simulink model "IB_BIEN_y_TG_BIEN"  (Simulink 8.1)
settings: Solver=ode45  StartTime=0.0  StopTime=50  RelTol=1e-3
PreLoadFcn:
  | Initial_datab
  | Const_IB
values from neighbouring files (symbols this model uses):
  a1 = (Iyy-Izz)/Ixx    (= -1.125)    [Initial_datab.m]
  a2 = Jr/Ixx    (= 0.00697115384615)    [Initial_datab.m]
  a3 = (Izz-Ixx)/Iyy    (= 1.11607142857)    [Initial_datab.m]
  a5 = (Ixx-Iyy)/Izz    (= -0.0349344978166)    [Initial_datab.m]
  alp1 = 20    [Initial_datab.m]
  alp2 = 10    [Initial_datab.m]
  b = 1.2*10^(-4)    (= 0.00012)    [Initial_datab.m]
  b1 = 1/Ixx    (= 96.1538461538)    [Initial_datab.m]
  b2 = 1/Iyy    (= 89.2857142857)    [Initial_datab.m]
  b3 = 1/Izz    (= 43.6681222707)    [Initial_datab.m]
  c1 = 10    [Const_IB.m]
  c10 = 0.75    [Const_IB.m]
  c11 = 1    [Const_IB.m]
  c12 = 0.75    [Const_IB.m]
  c2 = 6    [Const_IB.m]
  c3 = 10    [Const_IB.m]
  c4 = 6    [Const_IB.m]
  c5 = 2    [Const_IB.m]
  c6 = 2    [Const_IB.m]
  c7 = 3.5    [Const_IB.m]
  c8 = 1.5    [Const_IB.m]
  c9 = 1    [Const_IB.m]
  d = 3*10^(-6)    (= 3e-06)    [Initial_datab.m]
  Ixx = 10.4*10^(-3)    (= 0.0104)    [Initial_datab.m]
  Iyy = 11.2*10^(-3)    (= 0.0112)    [Initial_datab.m]
  Izz = 2.29*10^(-2)    (= 0.0229)    [Initial_datab.m]
  Jr = 7.25*10^(-5)    (= 7.25e-05)    [Initial_datab.m]
  k1x = -k1x    (= -0.5)    [Initial_datab.m]
  k1y = -k1y    (= -0.5)    [Initial_datab.m]
  k1z = -k1z    (= -2)    [Initial_datab.m]
  l = 0.225    [Initial_datab.m]
  ld1 = 0.07    [Const_IB.m]
  ld2 = 0.05    [Const_IB.m]
  ld3 = 0.01    [Const_IB.m]
  ld4 = 0.01    [Const_IB.m]
  ld5 = 0.001    [Const_IB.m]
  ld6 = 0.001    [Const_IB.m]
  m = 1.14    [Initial_datab.m]
  phi0 = 0    [Initial_datab.m]
  phi0dot = 0    [Initial_datab.m]
  psi0 = 0    [Initial_datab.m]
  psi0dot = 0    [Initial_datab.m]
  theta0 = 0    [Initial_datab.m]
  theta0dot = 0    [Initial_datab.m]
  x0 = 0    [Initial_datab.m]
  x0dot = 0    [Initial_datab.m]
  xf = -5    [Initial_datab.m]
  xfdot = 0    [Initial_datab.m]
  y0 = 0    [Initial_datab.m]
  y0dot = 0    [Initial_datab.m]
  yf = 5    [Initial_datab.m]
  yfdot = 0    [Initial_datab.m]
  z0 = 0    [Initial_datab.m]
  z0dot = 0    [Initial_datab.m]
  zf = 50    [Initial_datab.m]
  zfdot = 0    [Initial_datab.m]
undefined symbols (not defined in the file or in its folder): sigbuilder_block
(part 2 of 2)

== system IB_BIEN_y_TG_BIEN/TRAJECTORY GENERATION/Subsystem5/Subsystem1 ==
  t : Inport
  In2 : Inport  Port=2
  y_ent0 : Inport  Port=3
  Enabled Subsystem : Subsystem  TreatAsAtomicUnit=on
  Enabled Subsystem1 : Subsystem  TreatAsAtomicUnit=on
  Merge : Merge
  Relational Operator : RelationalOperator  Operator===  OutDataTypeStr=boolean
  Relational Operator1 : RelationalOperator  Operator=~=  OutDataTypeStr=boolean
  y0 : Outport
  wires:
  t/1 -> Relational Operator1/1, Relational Operator/1
  In2/1 -> Relational Operator/2, Relational Operator1/2, Enabled Subsystem1/1(In1)
  Relational Operator/1 -> Enabled Subsystem/Enable
  Enabled Subsystem/1(Out1) -> Merge/1
  Relational Operator1/1 -> Enabled Subsystem1/Enable
  Enabled Subsystem1/1(Out1) -> Merge/2
  y_ent0/1 -> Enabled Subsystem/1(In1)
  Merge/1 -> y0/1

== system IB_BIEN_y_TG_BIEN/TRAJECTORY GENERATION/Subsystem5/Subsystem2 ==
  t : Inport
  In2 : Inport  Port=2
  z_ent0 : Inport  Port=3
  Enabled Subsystem : Subsystem  TreatAsAtomicUnit=on
  Enabled Subsystem1 : Subsystem  TreatAsAtomicUnit=on
  Merge : Merge
  Relational Operator : RelationalOperator  Operator===  OutDataTypeStr=boolean
  Relational Operator1 : RelationalOperator  Operator=~=  OutDataTypeStr=boolean
  z0 : Outport
  wires:
  t/1 -> Relational Operator1/1, Relational Operator/1
  In2/1 -> Relational Operator/2, Relational Operator1/2, Enabled Subsystem1/1(In1)
  Relational Operator/1 -> Enabled Subsystem/Enable
  Enabled Subsystem/1(Out1) -> Merge/1
  Relational Operator1/1 -> Enabled Subsystem1/Enable
  Enabled Subsystem1/1(Out1) -> Merge/2
  z_ent0/1 -> Enabled Subsystem/1(In1)
  Merge/1 -> z0/1

== system IB_BIEN_y_TG_BIEN/TRAJECTORY GENERATION/X POSITION/Enabled Subsystem ==
  In1 : Inport
  Enable : EnablePort
  Fcn : Fcn  Expr=u(1)*u(2)+u(3)
  Out1 : Outport
  wires:
  In1/1 -> Fcn/1
  Fcn/1 -> Out1/1

== system IB_BIEN_y_TG_BIEN/TRAJECTORY GENERATION/X POSITION/Enabled Subsystem1 ==
  In1 : Inport
  Enable : EnablePort
  Fcn : Fcn  Expr=u(4)
  Out1 : Outport
  wires:
  In1/1 -> Fcn/1
  Fcn/1 -> Out1/1

== system IB_BIEN_y_TG_BIEN/TRAJECTORY GENERATION/X POSITION/Enabled Subsystem2 ==
  In1 : Inport
  Enable : EnablePort
  Fcn : Fcn  Expr=u(7)*(u(2)-u(5))+u(6)
  Out1 : Outport
  wires:
  In1/1 -> Fcn/1
  Fcn/1 -> Out1/1

== system IB_BIEN_y_TG_BIEN/TRAJECTORY GENERATION/X POSITION/Enabled Subsystem3 ==
  In1 : Inport
  Enable : EnablePort
  Fcn : Fcn  Expr=u(6)
  Out1 : Outport
  wires:
  In1/1 -> Fcn/1
  Fcn/1 -> Out1/1

== system IB_BIEN_y_TG_BIEN/TRAJECTORY GENERATION/X POSITION/Subsystem ==
  x0dot : Inport
  k1x : Inport  Port=2
  Vxmax : Inport  Port=3
  Add1 : Sum  Inputs=+-
  Divide : Product  Inputs=*/
  T1x : Outport
  wires:
  Vxmax/1 -> Add1/1  "Vxmax"
  Add1/1 -> Divide/1
  x0dot/1 -> Add1/2
  Divide/1 -> T1x/1  "T1"
  k1x/1 -> Divide/2

== system IB_BIEN_y_TG_BIEN/TRAJECTORY GENERATION/X POSITION/Subsystem1 ==
  deltax : Inport
  x0dot : Inport  Port=2
  k1x : Inport  Port=3
  xfdot : Inport  Port=4
  k2x : Inport  Port=5
  Vxmax : Inport  Port=6
  Add2 : Sum  Inputs=+--++
  Divide1 : Product  Inputs=*/
  Fcn : Fcn  Expr=((u(1)^2)-(u(2)^2))/(2*u(3)*u(1))
  Fcn1 : Fcn  Expr=(u(1)-u(2))/u(3)
  Fcn2 : Fcn  Expr=(u(1)-u(2))/u(3)
  Fcn3 : Fcn  Expr=((u(1)^2)-(u(2)^2))/(2*u(3)*u(1))
  Mux{,1..3} (4 alike) : Mux  Inputs=3
  Tx : Outport
  wires:
  Vxmax/1 -> Divide1/2, Mux/1, Mux1/1, Mux2/1, Mux3/1  "Vxmax"
  deltax/1 -> Divide1/1  "deltax"
  x0dot/1 -> Mux/2, Mux2/2
  k1x/1 -> Mux/3, Mux2/3
  Add2/1 -> Tx/1
  Divide1/1 -> Add2/1
  Mux/1 -> Fcn/1
  Fcn/1 -> Add2/2
  Mux1/1 -> Fcn1/1
  Fcn1/1 -> Add2/3
  Mux2/1 -> Fcn2/1
  Fcn2/1 -> Add2/4
  Mux3/1 -> Fcn3/1
  Fcn3/1 -> Add2/5
  xfdot/1 -> Mux1/2, Mux3/2
  k2x/1 -> Mux3/3, Mux1/3

== system IB_BIEN_y_TG_BIEN/TRAJECTORY GENERATION/X POSITION/Subsystem2 ==
  T : Inport
  xfdot : Inport  Port=2
  k2x : Inport  Port=3
  Vxmax : Inport  Port=4
  Add1 : Sum  Inputs=+-
  Add2 : Sum
  Display{1..4} (4 alike) : Display
  Divide : Product  Inputs=*/
  T2x : Outport
  wires:
  Vxmax/1 -> Add1/1, Display2/1  "Vxmax"
  Add1/1 -> Divide/1
  xfdot/1 -> Add1/2
  k2x/1 -> Divide/2, Display3/1
  Divide/1 -> Add2/1, Display1/1
  T/1 -> Add2/2, Display4/1
  Add2/1 -> T2x/1

== system IB_BIEN_y_TG_BIEN/TRAJECTORY GENERATION/X POSITION/Subsystem3 ==
  t : Inport
  T1 : Inport  Port=2
  T : Inport  Port=3
  T2 : Inport  Port=4
  Logical Operator : Logic  AllPortsSameDT=off  OutDataTypeStr=boolean
  Logical Operator1 : Logic  AllPortsSameDT=off  OutDataTypeStr=boolean
  Relational Operator : RelationalOperator  Operator=<  OutDataTypeStr=boolean
  Relational Operator1 : RelationalOperator  OutDataTypeStr=boolean
  Relational Operator2 : RelationalOperator  Operator=<  OutDataTypeStr=boolean
  Relational Operator3 : RelationalOperator  Operator=<  OutDataTypeStr=boolean
  Relational Operator4 : RelationalOperator  OutDataTypeStr=boolean
  Relational Operator5 : RelationalOperator  OutDataTypeStr=boolean
  Out1 : Outport
  Out2 : Outport  Port=2
  Out3 : Outport  Port=3
  Out4 : Outport  Port=4
  wires:
  T1/1 -> Relational Operator1/2, Relational Operator/2
  T2/1 -> Relational Operator4/2, Relational Operator2/2
  Relational Operator1/1 -> Logical Operator/1
  Relational Operator2/1 -> Logical Operator/2
  Relational Operator3/1 -> Logical Operator1/1
  Relational Operator4/1 -> Logical Operator1/2
  t/1 -> Relational Operator1/1, Relational Operator2/1, Relational Operator3/1, Relational Operator4/1, Relational Operator5/1, Relational Operator/1
  T/1 -> Relational Operator3/2, Relational Operator5/2
  Relational Operator/1 -> Out1/1
  Logical Operator/1 -> Out2/1
  Logical Operator1/1 -> Out3/1
  Relational Operator5/1 -> Out4/1

== system IB_BIEN_y_TG_BIEN/TRAJECTORY GENERATION/X POSITION/Subsystem5 ==
  t : Inport
  T : Inport  Port=2
  k1 : Inport  Port=3
  Fcn3 : Fcn  Expr=u(3)*(1-exp(-alp2*abs(u(1)-u(2))))
  Gain2 : Gain  Gain=-(1/4)
  Mux2 : Mux  Inputs=3
  k2xapro : Outport
  wires:
  Mux2/1 -> Fcn3/1
  Gain2/1 -> Mux2/3  "k2"
  t/1 -> Mux2/1
  T/1 -> Mux2/2
  k1/1 -> Gain2/1
  Fcn3/1 -> k2xapro/1  "k2x_apro"

== system IB_BIEN_y_TG_BIEN/TRAJECTORY GENERATION/Y POSITION/Enabled Subsystem ==
  In1 : Inport
  Enable : EnablePort
  Fcn : Fcn  Expr=u(1)*u(2)+u(3)
  Out1 : Outport
  wires:
  In1/1 -> Fcn/1
  Fcn/1 -> Out1/1

== system IB_BIEN_y_TG_BIEN/TRAJECTORY GENERATION/Y POSITION/Enabled Subsystem1 ==
  In1 : Inport
  Enable : EnablePort
  Fcn : Fcn  Expr=u(4)
  Out1 : Outport
  wires:
  In1/1 -> Fcn/1
  Fcn/1 -> Out1/1

== system IB_BIEN_y_TG_BIEN/TRAJECTORY GENERATION/Y POSITION/Enabled Subsystem2 ==
  In1 : Inport
  Enable : EnablePort
  Fcn : Fcn  Expr=u(7)*(u(2)-u(5))+u(6)
  Out1 : Outport
  wires:
  In1/1 -> Fcn/1
  Fcn/1 -> Out1/1

== system IB_BIEN_y_TG_BIEN/TRAJECTORY GENERATION/Y POSITION/Enabled Subsystem3 ==
  In1 : Inport
  Enable : EnablePort
  Fcn : Fcn  Expr=u(6)
  Out1 : Outport
  wires:
  In1/1 -> Fcn/1
  Fcn/1 -> Out1/1

== system IB_BIEN_y_TG_BIEN/TRAJECTORY GENERATION/Y POSITION/Subsystem ==
  y0dot : Inport
  k1y : Inport  Port=2
  Vymax : Inport  Port=3
  Add1 : Sum  Inputs=+-
  Divide : Product  Inputs=*/
  T1y : Outport
  wires:
  Vymax/1 -> Add1/1  "Vxmax"
  Add1/1 -> Divide/1
  y0dot/1 -> Add1/2
  Divide/1 -> T1y/1  "T1"
  k1y/1 -> Divide/2

== system IB_BIEN_y_TG_BIEN/TRAJECTORY GENERATION/Y POSITION/Subsystem1 ==
  yf : Inport
  y0 : Inport  Port=2
  y0dot : Inport  Port=3
  k1y : Inport  Port=4
  yfdot : Inport  Port=5
  k2y : Inport  Port=6
  Vymax : Inport  Port=7
  Add : Sum  Inputs=+-
  Add2 : Sum  Inputs=+--++
  Divide1 : Product  Inputs=*/
  Fcn : Fcn  Expr=((u(1)^2)-(u(2)^2))/(2*u(3)*u(1))
  Fcn1 : Fcn  Expr=(u(1)-u(2))/u(3)
  Fcn2 : Fcn  Expr=(u(1)-u(2))/u(3)
  Fcn3 : Fcn  Expr=((u(1)^2)-(u(2)^2))/(2*u(3)*u(1))
  Mux{,1..3} (4 alike) : Mux  Inputs=3
  Ty : Outport
  wires:
  Add/1 -> Divide1/1  "deltay"
  Vymax/1 -> Divide1/2, Mux/1, Mux1/1, Mux2/1, Mux3/1  "Vymax"
  yf/1 -> Add/1
  y0/1 -> Add/2
  y0dot/1 -> Mux/2, Mux2/2
  k1y/1 -> Mux/3, Mux2/3
  Add2/1 -> Ty/1
  Divide1/1 -> Add2/1
  Mux/1 -> Fcn/1
  Fcn/1 -> Add2/2
  Mux1/1 -> Fcn1/1
  Fcn1/1 -> Add2/3
  Mux2/1 -> Fcn2/1
  Fcn2/1 -> Add2/4
  Mux3/1 -> Fcn3/1
  Fcn3/1 -> Add2/5
  yfdot/1 -> Mux1/2, Mux3/2
  k2y/1 -> Mux3/3, Mux1/3

== system IB_BIEN_y_TG_BIEN/TRAJECTORY GENERATION/Y POSITION/Subsystem2 ==
  T : Inport
  yfdot : Inport  Port=2
  k2y : Inport  Port=3
  Vymax : Inport  Port=4
  Add1 : Sum  Inputs=+-
  Add2 : Sum
  Divide : Product  Inputs=*/
  T2y : Outport
  wires:
  Vymax/1 -> Add1/1  "Vymax"
  Add1/1 -> Divide/1
  yfdot/1 -> Add1/2
  k2y/1 -> Divide/2
  Divide/1 -> Add2/1
  T/1 -> Add2/2
  Add2/1 -> T2y/1

== system IB_BIEN_y_TG_BIEN/TRAJECTORY GENERATION/Y POSITION/Subsystem3 ==
  t : Inport
  T1 : Inport  Port=2
  T : Inport  Port=3
  T2 : Inport  Port=4
  Logical Operator : Logic  AllPortsSameDT=off  OutDataTypeStr=boolean
  Logical Operator1 : Logic  AllPortsSameDT=off  OutDataTypeStr=boolean
  Relational Operator : RelationalOperator  Operator=<  OutDataTypeStr=boolean
  Relational Operator1 : RelationalOperator  OutDataTypeStr=boolean
  Relational Operator2 : RelationalOperator  Operator=<  OutDataTypeStr=boolean
  Relational Operator3 : RelationalOperator  Operator=<  OutDataTypeStr=boolean
  Relational Operator4 : RelationalOperator  OutDataTypeStr=boolean
  Relational Operator5 : RelationalOperator  OutDataTypeStr=boolean
  Out1 : Outport
  Out2 : Outport  Port=2
  Out3 : Outport  Port=3
  Out4 : Outport  Port=4
  wires:
  T1/1 -> Relational Operator1/2, Relational Operator/2
  T2/1 -> Relational Operator4/2, Relational Operator2/2
  Relational Operator1/1 -> Logical Operator/1
  Relational Operator2/1 -> Logical Operator/2
  Relational Operator3/1 -> Logical Operator1/1
  Relational Operator4/1 -> Logical Operator1/2
  t/1 -> Relational Operator1/1, Relational Operator2/1, Relational Operator3/1, Relational Operator4/1, Relational Operator5/1, Relational Operator/1
  T/1 -> Relational Operator3/2, Relational Operator5/2
  Relational Operator/1 -> Out1/1
  Logical Operator/1 -> Out2/1
  Logical Operator1/1 -> Out3/1
  Relational Operator5/1 -> Out4/1

== system IB_BIEN_y_TG_BIEN/TRAJECTORY GENERATION/Z POSITION/Enabled Subsystem ==
  In1 : Inport
  Enable : EnablePort
  Fcn : Fcn  Expr=u(1)*u(2)+u(3)
  Out1 : Outport
  wires:
  In1/1 -> Fcn/1
  Fcn/1 -> Out1/1

== system IB_BIEN_y_TG_BIEN/TRAJECTORY GENERATION/Z POSITION/Enabled Subsystem1 ==
  In1 : Inport
  Enable : EnablePort
  Fcn : Fcn  Expr=u(4)
  Out1 : Outport
  wires:
  In1/1 -> Fcn/1
  Fcn/1 -> Out1/1

== system IB_BIEN_y_TG_BIEN/TRAJECTORY GENERATION/Z POSITION/Enabled Subsystem2 ==
  In1 : Inport
  Enable : EnablePort
  Fcn : Fcn  Expr=u(7)*(u(2)-u(5))+u(6)
  Out1 : Outport
  wires:
  In1/1 -> Fcn/1
  Fcn/1 -> Out1/1

== system IB_BIEN_y_TG_BIEN/TRAJECTORY GENERATION/Z POSITION/Enabled Subsystem3 ==
  In1 : Inport
  Enable : EnablePort
  Fcn : Fcn  Expr=u(6)
  Out1 : Outport
  wires:
  In1/1 -> Fcn/1
  Fcn/1 -> Out1/1

== system IB_BIEN_y_TG_BIEN/TRAJECTORY GENERATION/Z POSITION/Subsystem ==
  z0dot : Inport
  k1z : Inport  Port=2
  Vzmax : Inport  Port=3
  Add1 : Sum  Inputs=+-
  Divide : Product  Inputs=*/
  T1 : Outport
  wires:
  Vzmax/1 -> Add1/1  "Vxmax"
  Add1/1 -> Divide/1
  z0dot/1 -> Add1/2
  Divide/1 -> T1/1  "T1"
  k1z/1 -> Divide/2

== system IB_BIEN_y_TG_BIEN/TRAJECTORY GENERATION/Z POSITION/Subsystem1 ==
  zf : Inport
  z0 : Inport  Port=2
  z0dot : Inport  Port=3
  k1z : Inport  Port=4
  zfdot : Inport  Port=5
  k2z : Inport  Port=6
  Vzmax : Inport  Port=7
  Add : Sum  Inputs=+-
  Add2 : Sum  Inputs=+--++
  Divide1 : Product  Inputs=*/
  Fcn : Fcn  Expr=((u(1)^2)-(u(2)^2))/(2*u(3)*u(1))
  Fcn1 : Fcn  Expr=(u(1)-u(2))/u(3)
  Fcn2 : Fcn  Expr=(u(1)-u(2))/u(3)
  Fcn3 : Fcn  Expr=((u(1)^2)-(u(2)^2))/(2*u(3)*u(1))
  Mux{,1..3} (4 alike) : Mux  Inputs=3
  T : Outport
  wires:
  Add/1 -> Divide1/1  "deltaz"
  zf/1 -> Add/1
  z0/1 -> Add/2
  z0dot/1 -> Mux/2, Mux2/2
  k1z/1 -> Mux/3, Mux2/3
  Add2/1 -> T/1
  Divide1/1 -> Add2/1
  Mux/1 -> Fcn/1
  Fcn/1 -> Add2/2
  Mux1/1 -> Fcn1/1
  Fcn1/1 -> Add2/3
  Mux2/1 -> Fcn2/1
  Fcn2/1 -> Add2/4
  Mux3/1 -> Fcn3/1
  Fcn3/1 -> Add2/5
  zfdot/1 -> Mux1/2, Mux3/2
  k2z/1 -> Mux3/3, Mux1/3
  Vzmax/1 -> Divide1/2, Mux/1, Mux1/1, Mux2/1, Mux3/1  "Vzmax"

== system IB_BIEN_y_TG_BIEN/TRAJECTORY GENERATION/Z POSITION/Subsystem2 ==
  T : Inport
  zfdot : Inport  Port=2
  k2z : Inport  Port=3
  Vzmax : Inport  Port=4
  Add1 : Sum  Inputs=+-
  Add2 : Sum
  Divide : Product  Inputs=*/
  T2 : Outport
  wires:
  Vzmax/1 -> Add1/1  "Vzmax"
  Add1/1 -> Divide/1
  zfdot/1 -> Add1/2
  k2z/1 -> Divide/2
  Divide/1 -> Add2/1
  T/1 -> Add2/2
  Add2/1 -> T2/1

== system IB_BIEN_y_TG_BIEN/TRAJECTORY GENERATION/Z POSITION/Subsystem3 ==
  t : Inport
  T1 : Inport  Port=2
  T : Inport  Port=3
  T2 : Inport  Port=4
  Logical Operator : Logic  AllPortsSameDT=off  OutDataTypeStr=boolean
  Logical Operator1 : Logic  AllPortsSameDT=off  OutDataTypeStr=boolean
  Relational Operator : RelationalOperator  Operator=<  OutDataTypeStr=boolean
  Relational Operator1 : RelationalOperator  OutDataTypeStr=boolean
  Relational Operator2 : RelationalOperator  Operator=<  OutDataTypeStr=boolean
  Relational Operator3 : RelationalOperator  Operator=<  OutDataTypeStr=boolean
  Relational Operator4 : RelationalOperator  OutDataTypeStr=boolean
  Relational Operator5 : RelationalOperator  OutDataTypeStr=boolean
  Out1 : Outport
  Out2 : Outport  Port=2
  Out3 : Outport  Port=3
  Out4 : Outport  Port=4
  wires:
  T1/1 -> Relational Operator1/2, Relational Operator/2
  T2/1 -> Relational Operator4/2, Relational Operator2/2
  Relational Operator1/1 -> Logical Operator/1
  Relational Operator2/1 -> Logical Operator/2
  Relational Operator3/1 -> Logical Operator1/1
  Relational Operator4/1 -> Logical Operator1/2
  t/1 -> Relational Operator1/1, Relational Operator2/1, Relational Operator3/1, Relational Operator4/1, Relational Operator5/1, Relational Operator/1
  T/1 -> Relational Operator3/2, Relational Operator5/2
  Relational Operator/1 -> Out1/1
  Logical Operator/1 -> Out2/1
  Logical Operator1/1 -> Out3/1
  Relational Operator5/1 -> Out4/1

== system IB_BIEN_y_TG_BIEN/TRAJECTORY GENERATION/Subsystem5/Subsystem/Enabled Subsystem ==
  In1 : Inport
  Enable : EnablePort
  Out1 : Outport
  wires:
  In1/1 -> Out1/1

== system IB_BIEN_y_TG_BIEN/TRAJECTORY GENERATION/Subsystem5/Subsystem/Enabled Subsystem1 ==
  In1 : Inport
  Enable : EnablePort
  Out1 : Outport
  wires:
  In1/1 -> Out1/1

== system IB_BIEN_y_TG_BIEN/TRAJECTORY GENERATION/Subsystem5/Subsystem1/Enabled Subsystem ==
  In1 : Inport
  Enable : EnablePort
  Out1 : Outport
  wires:
  In1/1 -> Out1/1

== system IB_BIEN_y_TG_BIEN/TRAJECTORY GENERATION/Subsystem5/Subsystem1/Enabled Subsystem1 ==
  In1 : Inport
  Enable : EnablePort
  Out1 : Outport
  wires:
  In1/1 -> Out1/1

== system IB_BIEN_y_TG_BIEN/TRAJECTORY GENERATION/Subsystem5/Subsystem2/Enabled Subsystem ==
  In1 : Inport
  Enable : EnablePort
  Out1 : Outport
  wires:
  In1/1 -> Out1/1

== system IB_BIEN_y_TG_BIEN/TRAJECTORY GENERATION/Subsystem5/Subsystem2/Enabled Subsystem1 ==
  In1 : Inport
  Enable : EnablePort
  Out1 : Outport
  wires:
  In1/1 -> Out1/1
